simulink model "ACCDriver"  (R2017b)
settings: Solver=VariableStepAuto  StartTime=0.0  StopTime=10.0  RelTol=1e-3
undefined symbols (not defined in the file): default_spacing, Ki, Kp, max_ac, min_ac, time_gap, Ts, v_set, verr_gain, vx_gain, xerr_gain
libraries: autolibsharedcommon x3, autolibshared x1
settings Model: Creator=tacrain  LastModifiedBy=tacrain

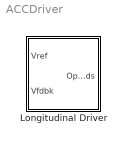
== system ACCDriver ==
  Longitudinal Driver : Subsystem
      mask Display: image('LongitudinalDriver.png', 'center')

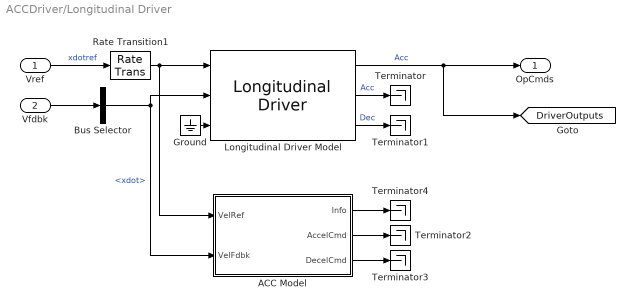
== system ACCDriver/Longitudinal Driver ==
  Vref : Inport
  Vfdbk : Inport  Port=2
  ACC Model : Subsystem
  Bus Selector : BusSelector  OutputSignals=Veh.xdot
  Ground : Ground
  Longitudinal Driver Model : autolibshared/Longitudinal Driver  vnom=5  Kp=1.5  Ki=1.5  Kaw=1  Kff=.1  Kg=0  tauerr=0.01
      settings: SourceProductName=Powertrain Blockset  SourceProductBaseCode=PW
  Rate Transition1 : RateTransition
  Terminator{,1..4} (5 alike) : Terminator
  OpCmds : Outport
  tag scope: DriverOutputs=global
  wires:
  Bus Selector/1 -> ACC Model/2(VelFdbk), Longitudinal Driver Model/2  "<xdot>"
  Vref/1 -> Rate Transition1/1  "xdotref"
  Vfdbk/1 -> Bus Selector/1
  Longitudinal Driver Model/1 -> [DriverOutputs], OpCmds/1  "Acc"
  Longitudinal Driver Model/2 -> Terminator/1  "Acc"
  Longitudinal Driver Model/3 -> Terminator1/1  "Dec"
  Ground/1 -> Longitudinal Driver Model/3
  Rate Transition1/1 -> ACC Model/1(VelRef), Longitudinal Driver Model/1
  ACC Model/2(AccelCmd) -> Terminator2/1
  ACC Model/3(DecelCmd) -> Terminator3/1
  ACC Model/1(Info) -> Terminator4/1

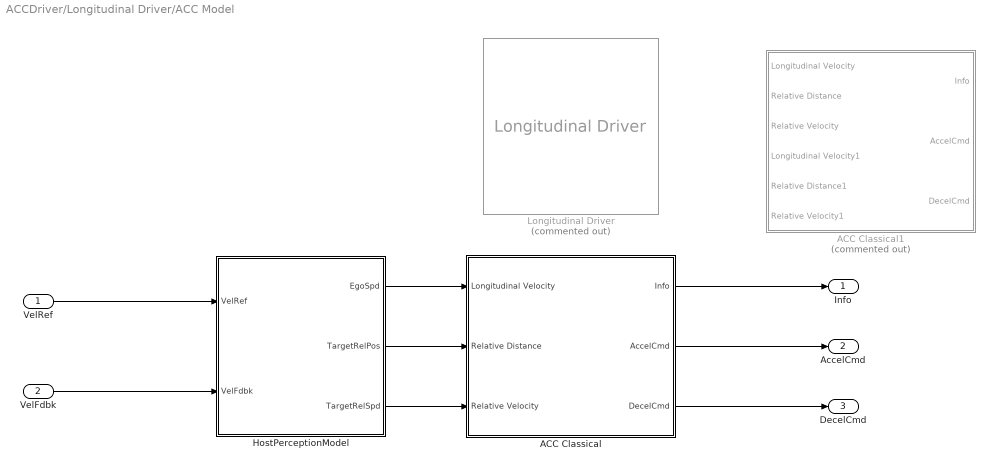
== system ACCDriver/Longitudinal Driver/ACC Model ==
  VelRef : Inport
  VelFdbk : Inport  Port=2
  ACC Classical : Subsystem  TreatAsAtomicUnit=on  VariantControl=controller_type == 1
      settings: RTWFileNameOpts=Use function name
  ACC Classical1 : Subsystem  Commented=on  TreatAsAtomicUnit=on  VariantControl=controller_type == 1
      settings: RTWFileNameOpts=Use function name
  HostPerceptionModel : Subsystem
  Longitudinal Driver : autolibsharedcommon/Longitudinal Driver  Commented=on  vnom=vnom  Kp=Kp  Ki=Ki  Kaw=Kaw  Kff=Kff  Kg=Kg  tauerr=tauerr
      settings: SourceProductName=Powertrain Blockset  SourceProductBaseCode=PW
  Info : Outport  InitialOutput=0
  AccelCmd : Outport  Port=2
  DecelCmd : Outport  Port=3
  wires:
  VelRef/1 -> HostPerceptionModel/1(VelRef)
  VelFdbk/1 -> HostPerceptionModel/2(VelFdbk)
  HostPerceptionModel/2(TargetRelPos) -> ACC Classical/2(Relative Distance)
  HostPerceptionModel/1(EgoSpd) -> ACC Classical/1(Longitudinal Velocity)
  HostPerceptionModel/3(TargetRelSpd) -> ACC Classical/3(Relative Velocity)
  ACC Classical/2(AccelCmd) -> AccelCmd/1
  ACC Classical/1(Info) -> Info/1
  ACC Classical/3(DecelCmd) -> DecelCmd/1

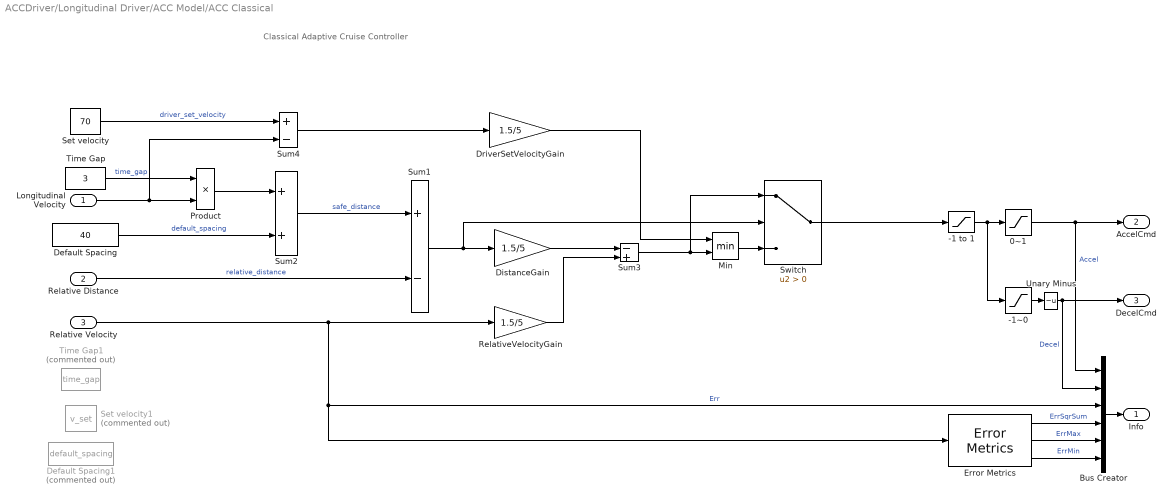
== system ACCDriver/Longitudinal Driver/ACC Model/ACC Classical ==
  note: Classical Adaptive Cruise Controller
  Longitudinal Velocity : Inport
  Relative Distance : Inport  Port=2
  Relative Velocity : Inport  Port=3
  " DistanceGain" : Gain  Gain=1.5/5
  " DriverSetVelocityGain" : Gain  Gain=1.5/5
  " RelativeVelocityGain" : Gain  Gain=1.5/5
  "-1 to 1 " : Saturate  UpperLimit=1  LowerLimit=-1
  -1~0 : Saturate  UpperLimit=0  LowerLimit=-1  ZeroCross=off
  0~1 : Saturate  UpperLimit=1  LowerLimit=0  ZeroCross=off
  Bus Creator : BusCreator  Inputs=6
  Default Spacing : Constant  Value=40  SampleTime=-1
  Default Spacing1 : Constant  Commented=on  Value=default_spacing  SampleTime=Ts
  Error Metrics : autolibsharedcommon/Longitudinal Driver/Error Metrics
      settings: SourceProductName=Powertrain Blockset  SourceProductBaseCode=PW
  Min : MinMax  Inputs=2
  Product : Product
  Set velocity : Constant  Value=70  SampleTime=-1
  Set velocity1 : Constant  Commented=on  Value=v_set  SampleTime=Ts
  Sum1 : Sum  Inputs=+-
  Sum2 : Sum
  Sum3 : Sum  Inputs=-+
  Sum4 : Sum  Inputs=+-
  Switch : Switch  Criteria=u2 > Threshold
  Time Gap : Constant  Value=3  SampleTime=-1
  Time Gap1 : Constant  Commented=on  Value=time_gap  SampleTime=Ts
  Unary Minus : UnaryMinus
  Info : Outport  InitialOutput=0
  AccelCmd : Outport  Port=2  Unit=one  InitialOutput=0
  DecelCmd : Outport  Port=3  Unit=one  InitialOutput=0
  wires:
  Longitudinal Velocity/1 -> Sum4/2, Product/2
  Default Spacing/1 -> Sum2/2  "default_spacing"
  " DistanceGain"/1 -> Sum3/1
  Sum4/1 -> " DriverSetVelocityGain"/1
  Min/1 -> Switch/3
  " RelativeVelocityGain"/1 -> Sum3/2
  Relative Velocity/1 -> Bus Creator/3, Error Metrics/1, " RelativeVelocityGain"/1  "Err"
  Time Gap/1 -> Product/1  "time_gap"
  Product/1 -> Sum2/1
  Sum2/1 -> Sum1/1  "safe_distance"
  Set velocity/1 -> Sum4/1  "driver_set_velocity"
  Sum3/1 -> Switch/1, Min/2
  Sum1/1 -> Switch/2, " DistanceGain"/1
  " DriverSetVelocityGain"/1 -> Min/1
  Relative Distance/1 -> Sum1/2  "relative_distance"
  0~1/1 -> Bus Creator/1, AccelCmd/1  "Accel"
  Switch/1 -> "-1 to 1 "/1
  "-1 to 1 "/1 -> -1~0/1, 0~1/1
  Unary Minus/1 -> DecelCmd/1, Bus Creator/2  "Decel"
  -1~0/1 -> Unary Minus/1
  Error Metrics/3 -> Bus Creator/6  "ErrMin"
  Bus Creator/1 -> Info/1
  Error Metrics/2 -> Bus Creator/5  "ErrMax"
  Error Metrics/1 -> Bus Creator/4  "ErrSqrSum"

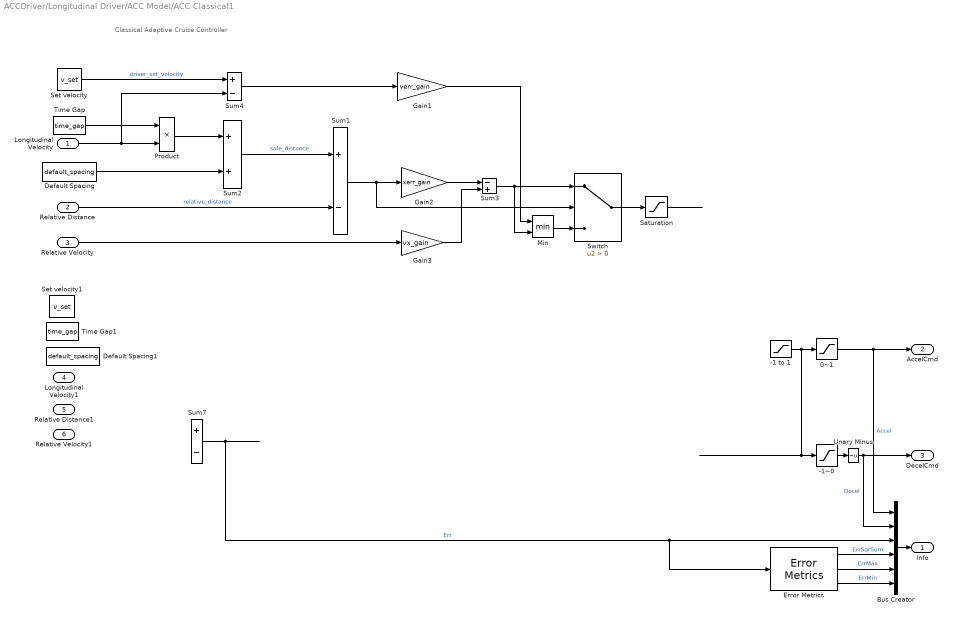
== system ACCDriver/Longitudinal Driver/ACC Model/ACC Classical1 ==
  note: Classical Adaptive Cruise Controller
  Longitudinal Velocity : Inport
  Relative Distance : Inport  Port=2
  Relative Velocity : Inport  Port=3
  Longitudinal Velocity1 : Inport  Port=4
  Relative Distance1 : Inport  Port=5
  Relative Velocity1 : Inport  Port=6
  "-1 to 1 " : Saturate  UpperLimit=1  LowerLimit=-1
  -1~0 : Saturate  UpperLimit=0  LowerLimit=-1  ZeroCross=off
  0~1 : Saturate  UpperLimit=1  LowerLimit=0  ZeroCross=off
  Bus Creator : BusCreator  Inputs=6
  Default Spacing : Constant  Value=default_spacing  SampleTime=Ts
  Default Spacing1 : Constant  Value=default_spacing  SampleTime=Ts
  Error Metrics : autolibsharedcommon/Longitudinal Driver/Error Metrics
      settings: SourceProductName=Powertrain Blockset  SourceProductBaseCode=PW
  Gain1 : Gain  Gain=verr_gain
  Gain2 : Gain  Gain=xerr_gain
  Gain3 : Gain  Gain=vx_gain
  Min : MinMax  Inputs=2
  Product : Product
  Saturation : Saturate  UpperLimit=max_ac  LowerLimit=min_ac
  Set velocity : Constant  Value=v_set  SampleTime=Ts
  Set velocity1 : Constant  Value=v_set  SampleTime=Ts
  Sum1 : Sum  Inputs=+-
  Sum2 : Sum
  Sum3 : Sum  Inputs=-+
  Sum4 : Sum  Inputs=+-
  Sum7 : Sum  Inputs=+-  SaturateOnIntegerOverflow=on  InputSameDT=on  OutDataTypeStr=Inherit: Same as first input
  Switch : Switch  Criteria=u2 > Threshold
  Time Gap : Constant  Value=time_gap  SampleTime=Ts
  Time Gap1 : Constant  Value=time_gap  SampleTime=Ts
  Unary Minus : UnaryMinus
  Info : Outport  InitialOutput=0
  AccelCmd : Outport  Port=2  Unit=one  InitialOutput=0
  DecelCmd : Outport  Port=3  Unit=one  InitialOutput=0
  wires:
  Sum7/1 -> Bus Creator/3, Error Metrics/1  "Err"
  Error Metrics/1 -> Bus Creator/4  "ErrSqrSum"
  Error Metrics/2 -> Bus Creator/5  "ErrMax"
  Bus Creator/1 -> Info/1
  Error Metrics/3 -> Bus Creator/6  "ErrMin"
  -1~0/1 -> Unary Minus/1
  Unary Minus/1 -> Bus Creator/2, DecelCmd/1  "Decel"
  "-1 to 1 "/1 -> 0~1/1, -1~0/1
  ? -> "-1 to 1 "/1
  0~1/1 -> AccelCmd/1, Bus Creator/1  "Accel"
  Relative Distance/1 -> Sum1/2  "relative_distance"
  Gain1/1 -> Min/1
  Sum1/1 -> Gain2/1, Switch/2
  Sum3/1 -> Switch/1, Min/2
  Set velocity/1 -> Sum4/1  "driver_set_velocity"
  Sum2/1 -> Sum1/1  "safe_distance"
  Product/1 -> Sum2/1
  Saturation/1 -> ?
  Time Gap/1 -> Product/1
  Relative Velocity/1 -> Gain3/1
  Switch/1 -> Saturation/1
  Gain3/1 -> Sum3/2
  Min/1 -> Switch/3
  Sum4/1 -> Gain1/1
  Gain2/1 -> Sum3/1
  Default Spacing/1 -> Sum2/2
  Longitudinal Velocity/1 -> Product/2, Sum4/2

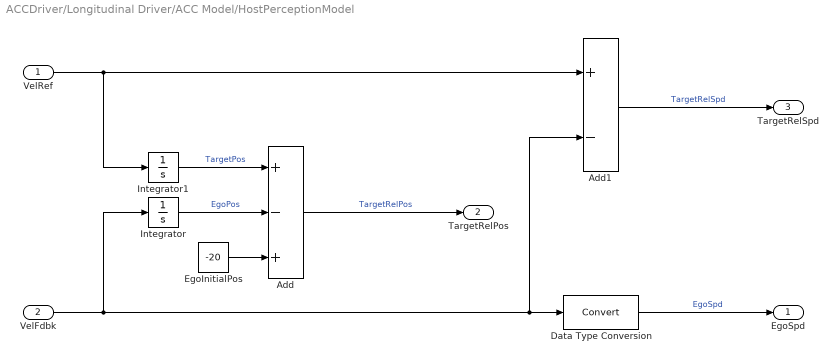
== system ACCDriver/Longitudinal Driver/ACC Model/HostPerceptionModel ==
  VelRef : Inport
  VelFdbk : Inport  Port=2
  Add : Sum  Inputs=+-+
  Add1 : Sum  Inputs=+-
  Data Type Conversion : DataTypeConversion
  EgoInitialPos : Constant  Value=-20
  Integrator : Integrator
  Integrator1 : Integrator
  EgoSpd : Outport
  TargetRelPos : Outport  Port=2
  TargetRelSpd : Outport  Port=3
  wires:
  VelRef/1 -> Integrator1/1, Add1/1
  EgoInitialPos/1 -> Add/3
  Add1/1 -> TargetRelSpd/1  "TargetRelSpd"
  Data Type Conversion/1 -> EgoSpd/1  "EgoSpd"
  Add/1 -> TargetRelPos/1  "TargetRelPos"
  Integrator/1 -> Add/2  "EgoPos"
  Integrator1/1 -> Add/1  "TargetPos"
  VelFdbk/1 -> Add1/2, Data Type Conversion/1, Integrator/1
